simulink model "CarritoDiferencial_tr"  (R2015a)
settings: Solver=ode4  StartTime=0.0  StopTime=50  FixedStep=.01  RelTol=1e-3
libraries: simulink x3
settings Model: Creator=Sala6  LastModifiedBy=Nicole

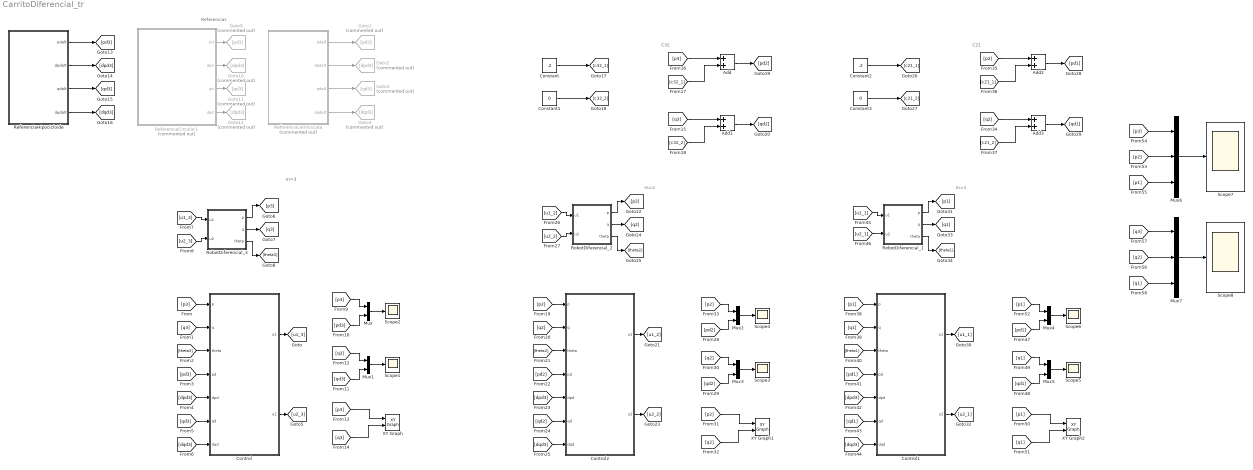
== system CarritoDiferencial_tr ==
  note: Referencias
  note: m=2
  note: C32
  note: m=3
  note: m=1
  note: C21
  Add{,1..3} (4 alike) : Sum
  Constant : Constant  Value=.2
  Constant1 : Constant  Value=0
  Constant2 : Constant  Value=.2
  Constant3 : Constant  Value=0
  Control : Subsystem  mask{kpp=200, kpq=200, rho=.1}
      mask prompts: kpp "Constante proporcional (kpp)"; kpq "Constante proporcional (kpq)"; rho "Excentricidad(rho)"
  Control1 : Subsystem  mask{kpp=200, kpq=200, rho=.1}
      mask prompts: kpp "Constante proporcional (kpp)"; kpq "Constante proporcional (kpq)"; rho "Excentricidad(rho)"
  Control2 : Subsystem  mask{kpp=200, kpq=200, rho=.1}
      mask prompts: kpp "Constante proporcional (kpp)"; kpq "Constante proporcional (kpq)"; rho "Excentricidad(rho)"
  Goto1 : Goto  Commented=on  GotoTag=pd3
  Goto10 : Goto  Commented=on  GotoTag=dpd3
  Goto11 : Goto  Commented=on  GotoTag=qd3
  Goto12 : Goto  Commented=on  GotoTag=dqd3
  Goto2 : Goto  Commented=on  GotoTag=dpd3
  Goto3 : Goto  Commented=on  GotoTag=qd3
  Goto4 : Goto  Commented=on  GotoTag=dqd3
  Goto9 : Goto  Commented=on  GotoTag=pd3
  Mux{,1..5} (6 alike) : Mux  Inputs=2
  Mux6 : Mux  Inputs=3
  Mux7 : Mux  Inputs=3
  ReferenciaCircular1 : Subsystem  Commented=on  mask{A=.5, w=pi/20}
      mask prompts: A "Radio"; w "Frecuencia"
  ReferenciaHipocicloide : Subsystem  mask{r=.05, k=10}
  ReferenciaLemniscata : Subsystem  Commented=on  mask{A=.5, w=pi/20}
      mask prompts: A "Radio"; w "Frecuencia"
  RobotDiferencial_1 : Subsystem  mask{p0=.25, q0=.1, theta0=0, rho=.1}
      mask prompts: p0 "Posicion inicial(p0)"; q0 "Posicion inicial(q0)"; theta0 "Orientacion inicial(theta0)"; rho "Excentricidad(rho)"
  RobotDiferencial_2 : Subsystem  mask{p0=.25, q0=.1, theta0=0, rho=.1}
      mask prompts: p0 "Posicion inicial(p0)"; q0 "Posicion inicial(q0)"; theta0 "Orientacion inicial(theta0)"; rho "Excentricidad(rho)"
  RobotDiferencial_3 : Subsystem  mask{p0=.2, q0=.4, theta0=0, rho=.1}
      mask prompts: p0 "Posicion inicial(p0)"; q0 "Posicion inicial(q0)"; theta0 "Orientacion inicial(theta0)"; rho "Excentricidad(rho)"
  Scope{1..8} (8 alike) : Scope
      Scope1 settings: TimeRange=auto  LimitDataPoints=on  MaxDataPoints=5000  SaveToWorkspace=off  YMin=-10  YMax=10  SampleTime=-1  DataFormat=Array
      Scope2 settings: TimeRange=auto  LimitDataPoints=on  MaxDataPoints=5000  SaveToWorkspace=off  SaveName=ScopeData  YMin=-12  YMax=12  SampleTime=-1  DataFormat=Array
      Scope3 settings: TimeRange=auto  LimitDataPoints=on  MaxDataPoints=5000  SaveToWorkspace=off  SaveName=ScopeData2  YMin=-10  YMax=10  SampleTime=-1  DataFormat=Array
      Scope4 settings: TimeRange=auto  LimitDataPoints=on  MaxDataPoints=5000  SaveToWorkspace=off  SaveName=ScopeData3  YMin=-12  YMax=12  SampleTime=-1  DataFormat=Array
      Scope5 settings: TimeRange=auto  LimitDataPoints=on  MaxDataPoints=5000  SaveToWorkspace=off  SaveName=ScopeData4  YMin=-10  YMax=10  SampleTime=-1  DataFormat=Array
      Scope6 settings: TimeRange=auto  LimitDataPoints=on  MaxDataPoints=5000  SaveToWorkspace=off  SaveName=ScopeData5  YMin=-12  YMax=12  SampleTime=-1  DataFormat=Array
      Scope7 settings: TimeRange=auto  LimitDataPoints=on  MaxDataPoints=5000  SaveName=p  YMin=-0.5  YMax=1  SampleTime=-1  DataFormat=Array
      Scope8 settings: TimeRange=auto  LimitDataPoints=on  MaxDataPoints=5000  SaveName=q  YMin=-0.625924  YMax=0.633259  SampleTime=-1  DataFormat=Array
  XY Graph : simulink/Sinks/XY Graph  xmin=-1  xmax=1  ymin=-1  ymax=1  st=-1
  XY Graph1 : simulink/Sinks/XY Graph  xmin=-1  xmax=1  ymin=-1  ymax=1  st=-1
  XY Graph2 : simulink/Sinks/XY Graph  xmin=-1  xmax=1  ymin=-1  ymax=1  st=-1
  wires:
  [p3] -> Control/1("p ")
  [q3] -> Control/2(q)
  [theta3] -> Control/3(theta)
  [pd3] -> Control/4(pd)
  [dpd3] -> Control/5(dpd)
  [qd3] -> Control/6(qd)
  [dqd3] -> Control/7(dqd)
  Control/1(u1) -> [u1_3]
  Control/2(u2) -> [u2_3]
  [u1_3] -> RobotDiferencial_3/1("u1 ")
  [u2_3] -> RobotDiferencial_3/2(u2)
  RobotDiferencial_3/1(p) -> [p3]
  RobotDiferencial_3/2(q) -> [q3]
  RobotDiferencial_3/3(theta) -> [theta3]
  Mux/1 -> Scope2/1
  [pd3] -> Mux/2
  [p3] -> Mux/1
  Mux1/1 -> Scope1/1
  [qd3] -> Mux1/2
  [q3] -> Mux1/1
  ReferenciaLemniscata/1(pdalt) -> Goto1/1
  ReferenciaLemniscata/2(dpdalt) -> Goto2/1
  ReferenciaLemniscata/3(qdalt) -> Goto3/1
  ReferenciaLemniscata/4(dqdalt) -> Goto4/1
  ReferenciaCircular1/1(pd) -> Goto9/1
  ReferenciaCircular1/2(dpd) -> Goto10/1
  ReferenciaCircular1/3(qd) -> Goto11/1
  ReferenciaCircular1/4("dqd ") -> Goto12/1
  ReferenciaHipocicloide/1(pdalt) -> [pd3]
  ReferenciaHipocicloide/2(dpdalt) -> [dpd3]
  ReferenciaHipocicloide/4(dqdalt) -> [dqd3]
  ReferenciaHipocicloide/3(qdalt) -> [qd3]
  [p3] -> XY Graph/1
  [q3] -> XY Graph/2
  Constant/1 -> [c32_1]
  Constant1/1 -> [c32_2]
  [p3] -> Add/1
  [c32_1] -> Add/2
  Add/1 -> [pd2]
  [q3] -> Add1/1
  [c32_2] -> Add1/2
  Add1/1 -> [qd2]
  [p2] -> Control2/1("p ")
  [q2] -> Control2/2(q)
  [theta2] -> Control2/3(theta)
  [pd2] -> Control2/4(pd)
  [dpd3] -> Control2/5(dpd)
  [qd2] -> Control2/6(qd)
  [dqd3] -> Control2/7(dqd)
  Control2/1(u1) -> [u1_2]
  Control2/2(u2) -> [u2_2]
  [u1_2] -> RobotDiferencial_2/1("u1 ")
  [u2_2] -> RobotDiferencial_2/2(u2)
  RobotDiferencial_2/1(p) -> [p2]
  RobotDiferencial_2/2(q) -> [q2]
  RobotDiferencial_2/3(theta) -> [theta2]
  Mux2/1 -> Scope4/1
  [pd2] -> Mux2/2
  [p2] -> Mux2/1
  Mux3/1 -> Scope3/1
  [qd2] -> Mux3/2
  [q2] -> Mux3/1
  [p2] -> XY Graph1/1
  [q2] -> XY Graph1/2
  Constant2/1 -> [c21_1]
  Constant3/1 -> [c21_2]
  [p2] -> Add2/1
  [c21_1] -> Add2/2
  Add2/1 -> [pd1]
  [q2] -> Add3/1
  [c21_2] -> Add3/2
  Add3/1 -> [qd1]
  [p1] -> Control1/1("p ")
  [q1] -> Control1/2(q)
  [theta1] -> Control1/3(theta)
  [pd1] -> Control1/4(pd)
  [dpd3] -> Control1/5(dpd)
  [qd1] -> Control1/6(qd)
  [dqd3] -> Control1/7(dqd)
  Control1/1(u1) -> [u1_1]
  Control1/2(u2) -> [u2_1]
  [u1_1] -> RobotDiferencial_1/1("u1 ")
  [u2_1] -> RobotDiferencial_1/2(u2)
  RobotDiferencial_1/1(p) -> [p1]
  RobotDiferencial_1/2(q) -> [q1]
  RobotDiferencial_1/3(theta) -> [theta1]
  Mux4/1 -> Scope6/1
  [pd1] -> Mux4/2
  [p1] -> Mux4/1
  Mux5/1 -> Scope5/1
  [qd1] -> Mux5/2
  [q1] -> Mux5/1
  [p1] -> XY Graph2/1
  [q1] -> XY Graph2/2
  Mux6/1 -> Scope7/1
  [p3] -> Mux6/1
  [p2] -> Mux6/2
  [p1] -> Mux6/3
  Mux7/1 -> Scope8/1
  [q3] -> Mux7/1
  [q2] -> Mux7/2
  [q1] -> Mux7/3

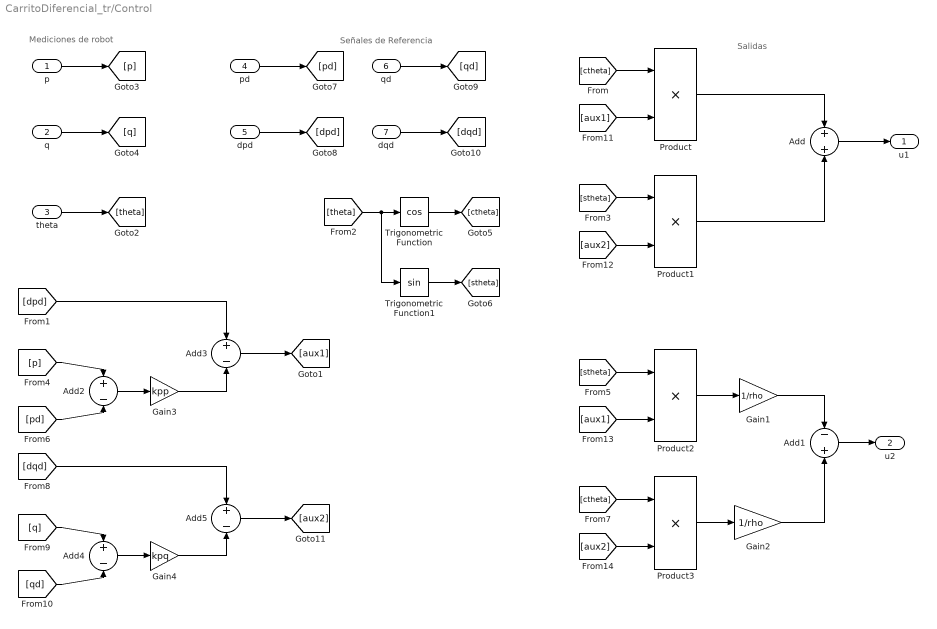
== system CarritoDiferencial_tr/Control ==
  note: Salidas
  note: Mediciones de robot
  note: Señales de Referencia
  "p " : Inport
  q : Inport  Port=2
  theta : Inport  Port=3
  pd : Inport  Port=4
  dpd : Inport  Port=5
  qd : Inport  Port=6
  dqd : Inport  Port=7
  Add : Sum
  Add1 : Sum  Inputs=-+
  Add{2..5} (4 alike) : Sum  Inputs=+-
  Gain1 : Gain  Gain=1/rho
  Gain2 : Gain  Gain=1/rho
  Gain3 : Gain  Gain=kpp
  Gain4 : Gain  Gain=kpq
  Product{,1..3} (4 alike) : Product
  Trigonometric Function : Trigonometry  Operator=cos
  Trigonometric Function1 : Trigonometry
  u1 : Outport
  u2 : Outport  Port=2
  wires:
  Gain2/1 -> Add1/2
  [stheta] -> Product2/1
  Product2/1 -> Gain1/1
  [ctheta] -> Product3/1
  Product3/1 -> Gain2/1
  Trigonometric Function/1 -> [ctheta]
  Product1/1 -> Add/2
  Product/1 -> Add/1
  q/1 -> [q]
  [stheta] -> Product1/1
  Trigonometric Function1/1 -> [stheta]
  [theta] -> Trigonometric Function/1, Trigonometric Function1/1
  "p "/1 -> [p]
  [ctheta] -> Product/1
  theta/1 -> [theta]
  pd/1 -> [pd]
  dpd/1 -> [dpd]
  qd/1 -> [qd]
  dqd/1 -> [dqd]
  [p] -> Add2/1
  [pd] -> Add2/2
  Add2/1 -> Gain3/1
  [dpd] -> Add3/1
  Gain3/1 -> Add3/2
  Add3/1 -> [aux1]
  [q] -> Add4/1
  [qd] -> Add4/2
  Add4/1 -> Gain4/1
  [dqd] -> Add5/1
  Gain4/1 -> Add5/2
  Add5/1 -> [aux2]
  [aux1] -> Product/2
  [aux2] -> Product1/2
  Add/1 -> u1/1
  Add1/1 -> u2/1
  Gain1/1 -> Add1/1
  [aux1] -> Product2/2
  [aux2] -> Product3/2

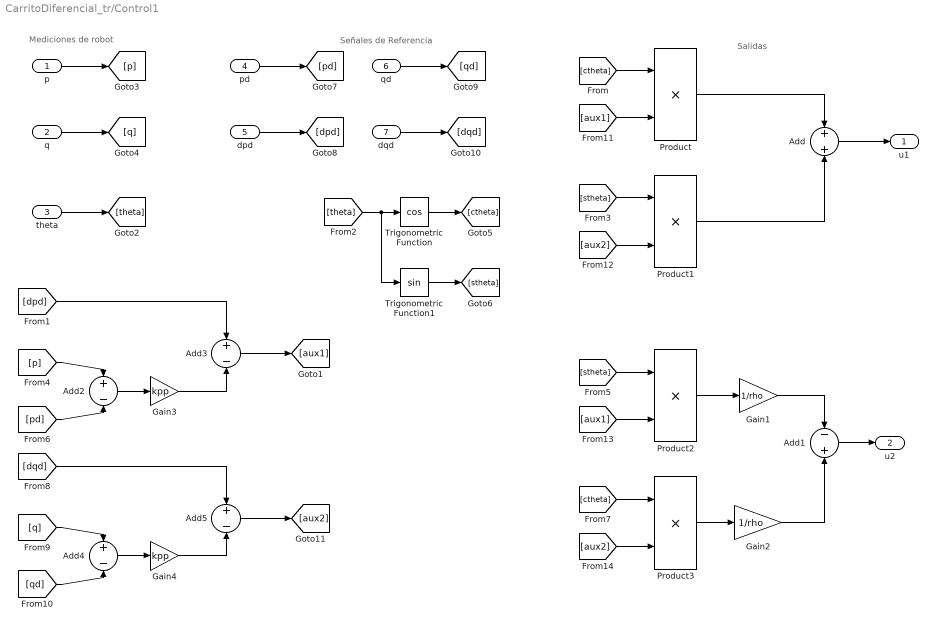
== system CarritoDiferencial_tr/Control1 ==
  note: Salidas
  note: Mediciones de robot
  note: Señales de Referencia
  "p " : Inport
  q : Inport  Port=2
  theta : Inport  Port=3
  pd : Inport  Port=4
  dpd : Inport  Port=5
  qd : Inport  Port=6
  dqd : Inport  Port=7
  Add : Sum
  Add1 : Sum  Inputs=-+
  Add{2..5} (4 alike) : Sum  Inputs=+-
  Gain1 : Gain  Gain=1/rho
  Gain2 : Gain  Gain=1/rho
  Gain3 : Gain  Gain=kpp
  Gain4 : Gain  Gain=kpp
  Product{,1..3} (4 alike) : Product
  Trigonometric Function : Trigonometry  Operator=cos
  Trigonometric Function1 : Trigonometry
  u1 : Outport
  u2 : Outport  Port=2
  wires:
  Gain2/1 -> Add1/2
  [stheta] -> Product2/1
  Product2/1 -> Gain1/1
  [ctheta] -> Product3/1
  Product3/1 -> Gain2/1
  Trigonometric Function/1 -> [ctheta]
  Product1/1 -> Add/2
  Product/1 -> Add/1
  q/1 -> [q]
  [stheta] -> Product1/1
  Trigonometric Function1/1 -> [stheta]
  [theta] -> Trigonometric Function/1, Trigonometric Function1/1
  "p "/1 -> [p]
  [ctheta] -> Product/1
  theta/1 -> [theta]
  pd/1 -> [pd]
  dpd/1 -> [dpd]
  qd/1 -> [qd]
  dqd/1 -> [dqd]
  [p] -> Add2/1
  [pd] -> Add2/2
  Add2/1 -> Gain3/1
  [dpd] -> Add3/1
  Gain3/1 -> Add3/2
  Add3/1 -> [aux1]
  [q] -> Add4/1
  [qd] -> Add4/2
  Add4/1 -> Gain4/1
  [dqd] -> Add5/1
  Gain4/1 -> Add5/2
  Add5/1 -> [aux2]
  [aux1] -> Product/2
  [aux2] -> Product1/2
  Add/1 -> u1/1
  Add1/1 -> u2/1
  Gain1/1 -> Add1/1
  [aux1] -> Product2/2
  [aux2] -> Product3/2

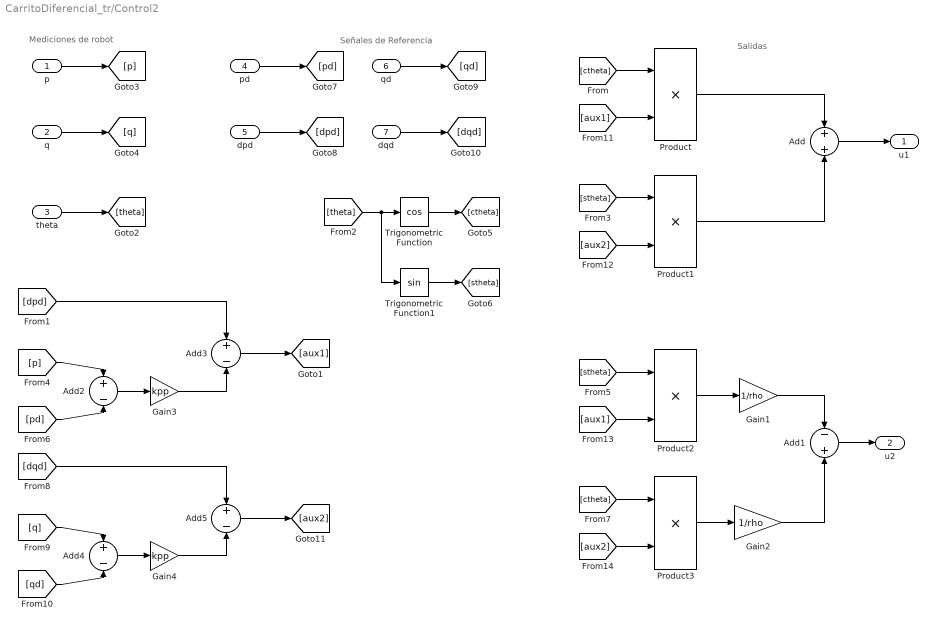
== system CarritoDiferencial_tr/Control2 ==
  note: Señales de Referencia
  note: Mediciones de robot
  note: Salidas
  "p " : Inport
  q : Inport  Port=2
  theta : Inport  Port=3
  pd : Inport  Port=4
  dpd : Inport  Port=5
  qd : Inport  Port=6
  dqd : Inport  Port=7
  Add : Sum
  Add1 : Sum  Inputs=-+
  Add{2..5} (4 alike) : Sum  Inputs=+-
  Gain1 : Gain  Gain=1/rho
  Gain2 : Gain  Gain=1/rho
  Gain3 : Gain  Gain=kpp
  Gain4 : Gain  Gain=kpp
  Product{,1..3} (4 alike) : Product
  Trigonometric Function : Trigonometry  Operator=cos
  Trigonometric Function1 : Trigonometry
  u1 : Outport
  u2 : Outport  Port=2
  wires:
  [aux2] -> Product3/2
  [aux1] -> Product2/2
  Gain1/1 -> Add1/1
  Add1/1 -> u2/1
  Add/1 -> u1/1
  [aux2] -> Product1/2
  [aux1] -> Product/2
  Add5/1 -> [aux2]
  Gain4/1 -> Add5/2
  [dqd] -> Add5/1
  Add4/1 -> Gain4/1
  [qd] -> Add4/2
  [q] -> Add4/1
  Add3/1 -> [aux1]
  Gain3/1 -> Add3/2
  [dpd] -> Add3/1
  Add2/1 -> Gain3/1
  [pd] -> Add2/2
  [p] -> Add2/1
  dqd/1 -> [dqd]
  qd/1 -> [qd]
  dpd/1 -> [dpd]
  pd/1 -> [pd]
  theta/1 -> [theta]
  [ctheta] -> Product/1
  "p "/1 -> [p]
  [theta] -> Trigonometric Function1/1, Trigonometric Function/1
  Trigonometric Function1/1 -> [stheta]
  [stheta] -> Product1/1
  q/1 -> [q]
  Product/1 -> Add/1
  Product1/1 -> Add/2
  Trigonometric Function/1 -> [ctheta]
  Product3/1 -> Gain2/1
  [ctheta] -> Product3/1
  Product2/1 -> Gain1/1
  [stheta] -> Product2/1
  Gain2/1 -> Add1/2

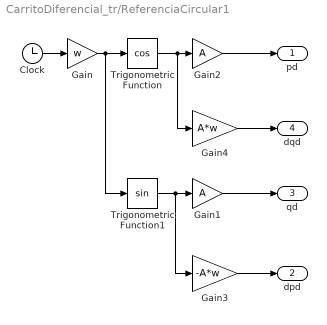
== system CarritoDiferencial_tr/ReferenciaCircular1 ==
  Clock : Clock
  Gain : Gain  Gain=w
  Gain1 : Gain  Gain=A
  Gain2 : Gain  Gain=A
  Gain3 : Gain  Gain=-A*w
  Gain4 : Gain  Gain=A*w
  Trigonometric Function : Trigonometry  Operator=cos
  Trigonometric Function1 : Trigonometry
  pd : Outport
  dpd : Outport  Port=2
  qd : Outport  Port=3
  "dqd " : Outport  Port=4
  wires:
  Gain4/1 -> "dqd "/1
  Gain3/1 -> dpd/1
  Trigonometric Function/1 -> Gain2/1, Gain4/1
  Gain/1 -> Trigonometric Function/1, Trigonometric Function1/1
  Gain1/1 -> qd/1
  Trigonometric Function1/1 -> Gain1/1, Gain3/1
  Clock/1 -> Gain/1
  Gain2/1 -> pd/1

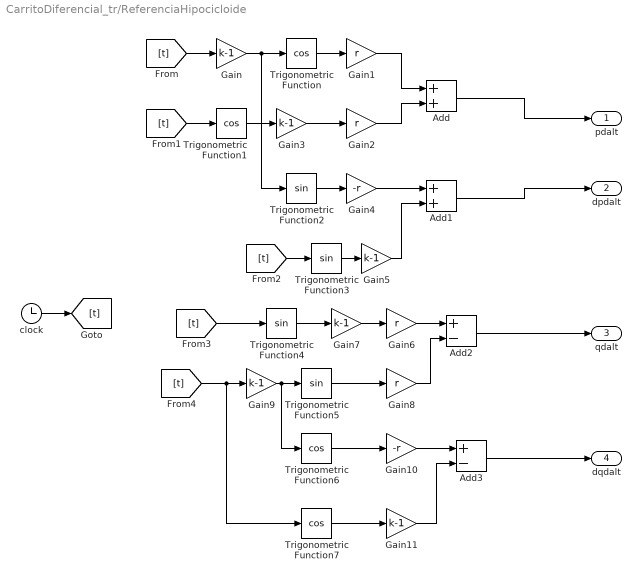
== system CarritoDiferencial_tr/ReferenciaHipocicloide ==
  Add : Sum
  Add1 : Sum
  Add2 : Sum  Inputs=+-
  Add3 : Sum  Inputs=+-
  Gain{,3,5,7,9,11} (6 alike) : Gain  Gain=k-1
  Gain{1..2,6,8} (4 alike) : Gain  Gain=r
  Gain10 : Gain  Gain=-r
  Gain4 : Gain  Gain=-r
  Trigonometric Function{,1,6..7} (4 alike) : Trigonometry  Operator=cos
  Trigonometric Function{2..5} (4 alike) : Trigonometry
  clock : Clock
  pdalt : Outport
  dpdalt : Outport  Port=2
  qdalt : Outport  Port=3
  dqdalt : Outport  Port=4
  wires:
  clock/1 -> [t]
  [t] -> Gain/1
  Gain/1 -> Trigonometric Function2/1, Trigonometric Function/1
  Trigonometric Function/1 -> Gain1/1
  Gain1/1 -> Add/1
  Trigonometric Function1/1 -> Gain3/1
  Gain2/1 -> Add/2
  [t] -> Trigonometric Function1/1
  Gain3/1 -> Gain2/1
  Add/1 -> pdalt/1
  Trigonometric Function2/1 -> Gain4/1
  Gain4/1 -> Add1/1
  Trigonometric Function3/1 -> Gain5/1
  [t] -> Trigonometric Function3/1
  Gain5/1 -> Add1/2
  Add1/1 -> dpdalt/1
  [t] -> Trigonometric Function4/1
  Gain7/1 -> Gain6/1
  Trigonometric Function4/1 -> Gain7/1
  Gain6/1 -> Add2/1
  Trigonometric Function5/1 -> Gain8/1
  [t] -> Trigonometric Function7/1, Gain9/1
  Gain8/1 -> Add2/2
  Add2/1 -> qdalt/1
  Trigonometric Function6/1 -> Gain10/1
  Gain9/1 -> Trigonometric Function6/1, Trigonometric Function5/1
  Gain10/1 -> Add3/1
  Add3/1 -> dqdalt/1
  Trigonometric Function7/1 -> Gain11/1
  Gain11/1 -> Add3/2

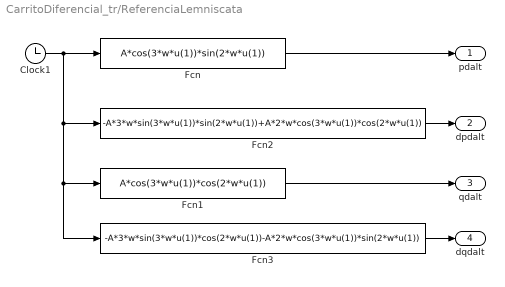
== system CarritoDiferencial_tr/ReferenciaLemniscata ==
  Clock1 : Clock
  Fcn : Fcn  Expr=A*cos(3*w*u(1))*sin(2*w*u(1))
  Fcn1 : Fcn  Expr=A*cos(3*w*u(1))*cos(2*w*u(1))
  Fcn2 : Fcn  Expr=-A*3*w*sin(3*w*u(1))*sin(2*w*u(1))+A*2*w*cos(3*w*u(1))*cos(2*w*u(1))
  Fcn3 : Fcn  Expr=-A*3*w*sin(3*w*u(1))*cos(2*w*u(1))-A*2*w*cos(3*w*u(1))*sin(2*w*u(1))
  pdalt : Outport
  dpdalt : Outport  Port=2
  qdalt : Outport  Port=3
  dqdalt : Outport  Port=4
  wires:
  Clock1/1 -> Fcn2/1, Fcn1/1, Fcn3/1, Fcn/1
  Fcn/1 -> pdalt/1
  Fcn2/1 -> dpdalt/1
  Fcn1/1 -> qdalt/1
  Fcn3/1 -> dqdalt/1

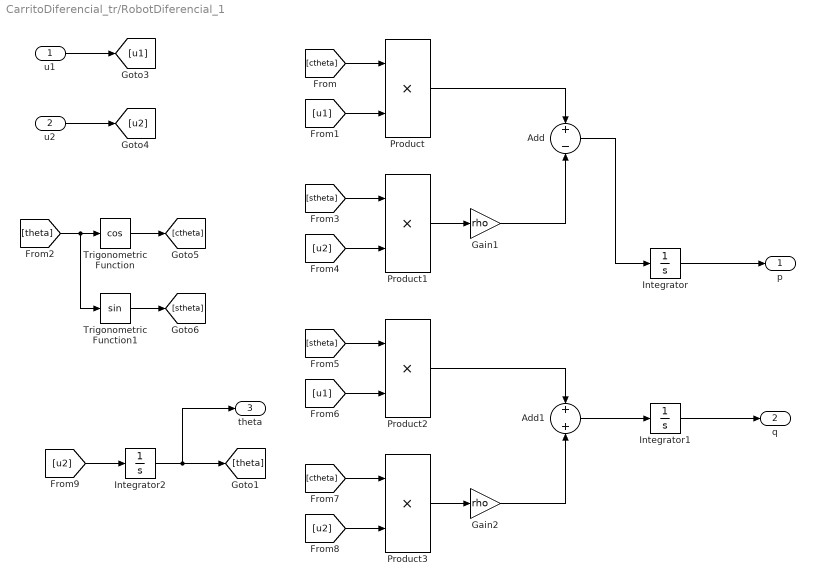
== system CarritoDiferencial_tr/RobotDiferencial_1 ==
  "u1 " : Inport
  u2 : Inport  Port=2
  Add : Sum  Inputs=+-
  Add1 : Sum
  Gain1 : Gain  Gain=rho
  Gain2 : Gain  Gain=rho
  Integrator : Integrator  InitialCondition=p0
  Integrator1 : Integrator  InitialCondition=q0
  Integrator2 : Integrator  InitialCondition=theta0
  Product{,1..3} (4 alike) : Product
  Trigonometric Function : Trigonometry  Operator=cos
  Trigonometric Function1 : Trigonometry
  p : Outport
  q : Outport  Port=2
  theta : Outport  Port=3
  wires:
  Integrator/1 -> p/1
  [ctheta] -> Product/1
  Integrator2/1 -> theta/1, [theta]
  Integrator1/1 -> q/1
  "u1 "/1 -> [u1]
  [theta] -> Trigonometric Function1/1, Trigonometric Function/1
  Trigonometric Function1/1 -> [stheta]
  Product1/1 -> Gain1/1
  [u2] -> Product1/2
  Add/1 -> Integrator/1
  [stheta] -> Product1/1
  [u1] -> Product/2
  u2/1 -> [u2]
  Product/1 -> Add/1
  Gain1/1 -> Add/2
  Trigonometric Function/1 -> [ctheta]
  Product3/1 -> Gain2/1
  [u2] -> Product3/2
  [u1] -> Product2/2
  [ctheta] -> Product3/1
  Product2/1 -> Add1/1
  [stheta] -> Product2/1
  Gain2/1 -> Add1/2
  [u2] -> Integrator2/1
  Add1/1 -> Integrator1/1

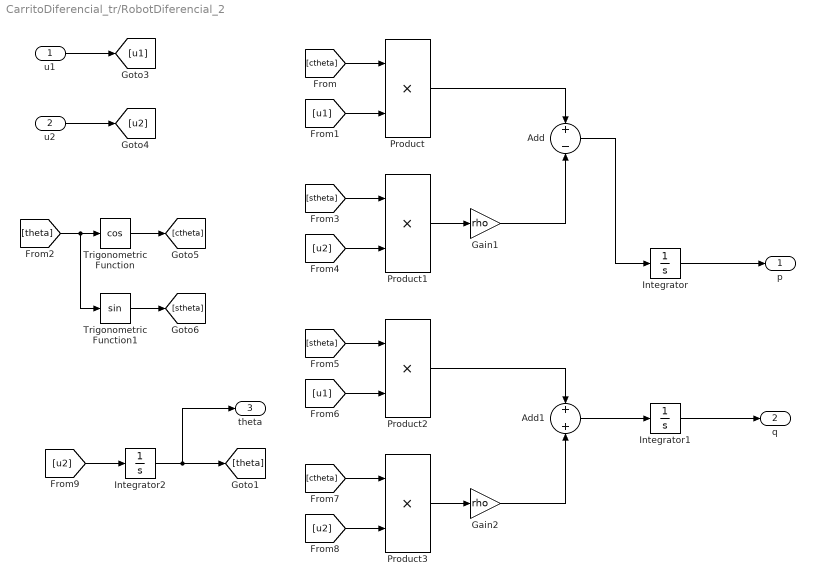
== system CarritoDiferencial_tr/RobotDiferencial_2 ==
  "u1 " : Inport
  u2 : Inport  Port=2
  Add : Sum  Inputs=+-
  Add1 : Sum
  Gain1 : Gain  Gain=rho
  Gain2 : Gain  Gain=rho
  Integrator : Integrator  InitialCondition=p0
  Integrator1 : Integrator  InitialCondition=q0
  Integrator2 : Integrator  InitialCondition=theta0
  Product{,1..3} (4 alike) : Product
  Trigonometric Function : Trigonometry  Operator=cos
  Trigonometric Function1 : Trigonometry
  p : Outport
  q : Outport  Port=2
  theta : Outport  Port=3
  wires:
  Add1/1 -> Integrator1/1
  [u2] -> Integrator2/1
  Gain2/1 -> Add1/2
  [stheta] -> Product2/1
  Product2/1 -> Add1/1
  [ctheta] -> Product3/1
  [u1] -> Product2/2
  [u2] -> Product3/2
  Product3/1 -> Gain2/1
  Trigonometric Function/1 -> [ctheta]
  Gain1/1 -> Add/2
  Product/1 -> Add/1
  u2/1 -> [u2]
  [u1] -> Product/2
  [stheta] -> Product1/1
  Add/1 -> Integrator/1
  [u2] -> Product1/2
  Product1/1 -> Gain1/1
  Trigonometric Function1/1 -> [stheta]
  [theta] -> Trigonometric Function/1, Trigonometric Function1/1
  "u1 "/1 -> [u1]
  Integrator1/1 -> q/1
  Integrator2/1 -> [theta], theta/1
  [ctheta] -> Product/1
  Integrator/1 -> p/1

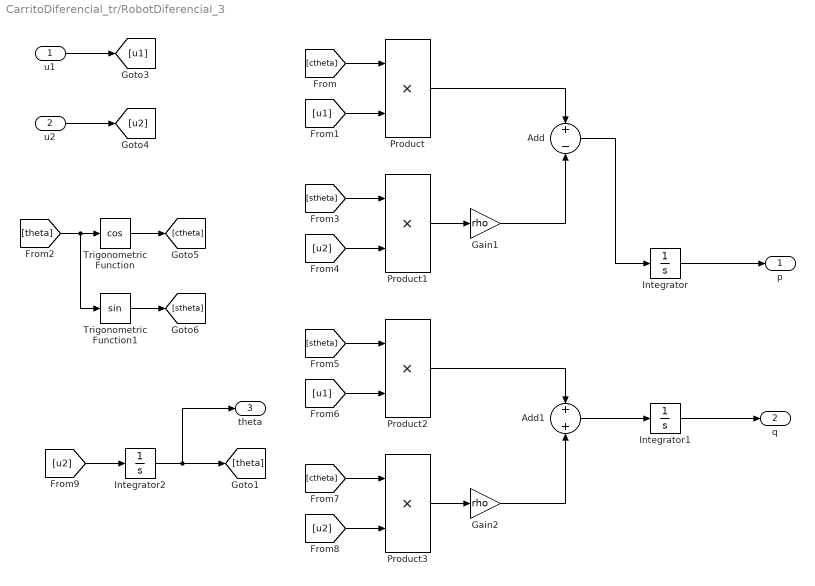
== system CarritoDiferencial_tr/RobotDiferencial_3 ==
  "u1 " : Inport
  u2 : Inport  Port=2
  Add : Sum  Inputs=+-
  Add1 : Sum
  Gain1 : Gain  Gain=rho
  Gain2 : Gain  Gain=rho
  Integrator : Integrator  InitialCondition=p0
  Integrator1 : Integrator  InitialCondition=q0
  Integrator2 : Integrator  InitialCondition=theta0
  Product{,1..3} (4 alike) : Product
  Trigonometric Function : Trigonometry  Operator=cos
  Trigonometric Function1 : Trigonometry
  p : Outport
  q : Outport  Port=2
  theta : Outport  Port=3
  wires:
  Integrator/1 -> p/1
  [ctheta] -> Product/1
  Integrator2/1 -> theta/1, [theta]
  Integrator1/1 -> q/1
  "u1 "/1 -> [u1]
  [theta] -> Trigonometric Function1/1, Trigonometric Function/1
  Trigonometric Function1/1 -> [stheta]
  Product1/1 -> Gain1/1
  [u2] -> Product1/2
  Add/1 -> Integrator/1
  [stheta] -> Product1/1
  [u1] -> Product/2
  u2/1 -> [u2]
  Product/1 -> Add/1
  Gain1/1 -> Add/2
  Trigonometric Function/1 -> [ctheta]
  Product3/1 -> Gain2/1
  [u2] -> Product3/2
  [u1] -> Product2/2
  [ctheta] -> Product3/1
  Product2/1 -> Add1/1
  [stheta] -> Product2/1
  Gain2/1 -> Add1/2
  [u2] -> Integrator2/1
  Add1/1 -> Integrator1/1
